simulink model "nls_col"  (Simulink 6.1)
settings: Solver=ode15s  SolverMode=SingleTasking  StartTime=0.0  StopTime=300  MaxStep=1  RelTol=1e-6  AbsTol=1e-6
values from neighbouring files (symbols this model uses):
  kf1 = 0.01/So(1,1)    [init_col.m]
  kf2 = 0.01/So(2,2)    [init_col.m]
  Tf11 = 1    [init_col.m]
  Tf12 = 1    [init_col.m]
  Tf21 = 1    [init_col.m]
  Tf22 = 1    [init_col.m]
undefined symbols (not defined in the file or in its folder): Ak, Bk, Ck, Dk
libraries: simulink x2
settings Model: LastModifiedBy=Petko Petkov
settings DataIOCC: LimitDataPoints=off  SaveOutput=off  SaveTime=off
settings OptimizationCC: BooleanDataType=off
settings HardwareCC: TargetUnknown=on
settings RTWCC: TemplateMakefile=grt_unix.tmf
settings GRTTargetCC: ModelReferenceCompliant=off  MatFileLogging=off

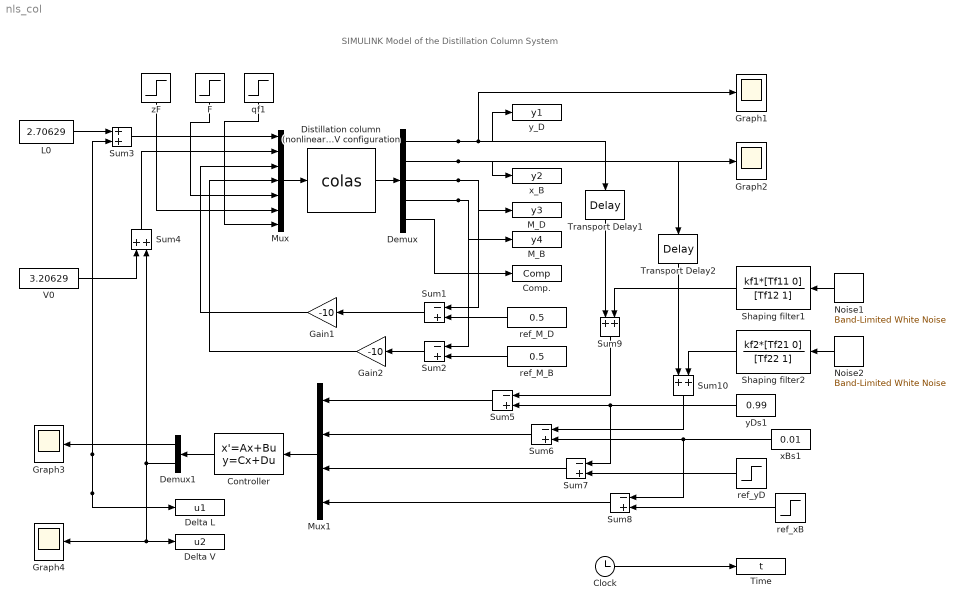
== system nls_col ==
  note: SIMULINK Model of the Distillation Column System
  Clock : Clock
      settings: Decimation=10
  Comp. : ToWorkspace  VariableName=Comp  SaveFormat=Array
      settings: MaxDataPoints=20000
  Controller : StateSpace  Orientation=left  A=Ak  B=Bk  C=Ck  D=Dk
  Delta L : ToWorkspace  VariableName=u1  SaveFormat=Array
      settings: MaxDataPoints=20000
  Delta V : ToWorkspace  VariableName=u2  SaveFormat=Array
      settings: MaxDataPoints=20000
  Demux : Demux  Outputs=5
  Demux1 : Demux  Orientation=left  Outputs=2
  Distillation column (nonlinear)  LV configuration : S-Function  FunctionName=colas
  F : Step  Orientation=down  Time=10  Before=1  After=1.2  SampleTime=0
  Gain1 : Gain  Orientation=left  Gain=-10  SaturateOnIntegerOverflow=on
  Gain2 : Gain  Orientation=left  Gain=-10  SaturateOnIntegerOverflow=on
  Graph{1..4} (4 alike) : Scope
      Graph1 settings: TickLabels=on  TimeRange=150  YMin=0.9895  YMax=0.995  DataFormat=Array  MaxDataPoints=20000
      Graph2 settings: TickLabels=on  TimeRange=20  YMin=-0.0065495  YMax=-0.00654525  DataFormat=Array  MaxDataPoints=20000
      Graph3 settings: TickLabels=on  TimeRange=150  YMin=0.985  YMax=1  SaveName=ScopeData2  DataFormat=Array  MaxDataPoints=20000
      Graph4 settings: TickLabels=on  TimeRange=150  YMin=0.985  YMax=1  DataFormat=Array  MaxDataPoints=20000
  L0 : Constant  Value=2.70629
  M_B : ToWorkspace  VariableName=y4  SaveFormat=Array
      settings: MaxDataPoints=20000
  M_D : ToWorkspace  VariableName=y3  SaveFormat=Array
      settings: MaxDataPoints=20000
  Mux : Mux  Inputs=7
  Mux1 : Mux  Orientation=left
  Noise1 : simulink/Sources/Band-Limited White Noise  Orientation=left  Cov=5*10^(-3)  Ts=1  seed=[23341]
  Noise2 : simulink/Sources/Band-Limited White Noise  Orientation=left  Cov=5*10^(-3)  Ts=1  seed=[23341]
  Shaping filter1 : TransferFcn  Orientation=left  Numerator=kf1*[Tf11 0]  Denominator=[Tf12 1]
  Shaping filter2 : TransferFcn  Orientation=left  Numerator=kf2*[Tf21 0]  Denominator=[Tf22 1]
  Sum{1..2,5..8} (6 alike) : Sum  Orientation=left  Inputs=-+  SaturateOnIntegerOverflow=on  InputSameDT=on
  Sum10 : Sum  Orientation=down  SaturateOnIntegerOverflow=on  InputSameDT=on
  Sum3 : Sum  SaturateOnIntegerOverflow=on  InputSameDT=on
  Sum4 : Sum  Orientation=up  SaturateOnIntegerOverflow=on  InputSameDT=on
  Sum9 : Sum  Orientation=down  SaturateOnIntegerOverflow=on  InputSameDT=on
  Time : ToWorkspace  VariableName=t  SaveFormat=Array
      settings: MaxDataPoints=20000
  Transport Delay1 : TransportDelay  Orientation=down  InitialInput=0.99
  Transport Delay2 : TransportDelay  Orientation=down  InitialInput=0.01
  V0 : Constant  Value=3.20629
  qf1 : Step  Orientation=down  Time=0  SampleTime=0
  ref_M_B : Constant  Orientation=left  Value=0.5
  ref_M_D : Constant  Orientation=left  Value=0.5
  ref_xB : Step  Orientation=left  Time=0  After=0.01  SampleTime=0
  ref_yD : Step  Orientation=left  Time=200  Before=0.99  After=0.995  SampleTime=0
  xBs1 : Constant  Orientation=left  Value=0.01
  x_B : ToWorkspace  VariableName=y2  SaveFormat=Array
      settings: MaxDataPoints=20000
  yDs1 : Constant  Orientation=left  Value=0.99
  y_D : ToWorkspace  VariableName=y1  SaveFormat=Array
      settings: MaxDataPoints=20000
  zF : Step  Orientation=down  Time=100  Before=0.5  After=0.6  SampleTime=0
  wires:
  V0/1 -> Sum4/1
  L0/1 -> Sum3/1
  qf1/1 -> Mux/7
  Gain2/1 -> Mux/4
  Sum2/1 -> Gain2/1
  ref_M_B/1 -> Sum2/2
  Gain1/1 -> Mux/3
  Mux/1 -> Distillation column (nonlinear)  LV configuration/1
  Distillation column (nonlinear)  LV configuration/1 -> Demux/1
  Clock/1 -> Time/1
  zF/1 -> Mux/6
  F/1 -> Mux/5
  Demux1/2 -> Sum4/2, Delta V/1, Graph4/1
  Demux1/1 -> Delta L/1, Graph3/1, Sum3/2
  Sum4/1 -> Mux/2
  Sum3/1 -> Mux/1
  Demux/1 -> Transport Delay1/1, y_D/1, Graph1/1
  Demux/2 -> Transport Delay2/1, Graph2/1, x_B/1
  Demux/3 -> Sum1/1, M_D/1
  Demux/4 -> Sum2/1, M_B/1
  Demux/5 -> Comp./1
  Controller/1 -> Demux1/1
  Sum6/1 -> Mux1/2
  Sum5/1 -> Mux1/1
  yDs1/1 -> Sum5/2, Sum7/1
  xBs1/1 -> Sum6/2, Sum8/1
  Mux1/1 -> Controller/1
  Sum7/1 -> Mux1/3
  Sum8/1 -> Mux1/4
  ref_yD/1 -> Sum7/2
  ref_xB/1 -> Sum8/2
  ref_M_D/1 -> Sum1/2
  Sum1/1 -> Gain1/1
  Sum9/1 -> Sum5/1
  Transport Delay1/1 -> Sum9/1
  Sum10/1 -> Sum6/1
  Transport Delay2/1 -> Sum10/1
  Noise1/1 -> Shaping filter1/1
  Shaping filter1/1 -> Sum9/2
  Noise2/1 -> Shaping filter2/1
  Shaping filter2/1 -> Sum10/2
